simulink model "SEDC_Motor_model"  (R2021a)
settings: Solver=VariableStepAuto  StartTime=0.0  StopTime=inf  MaxStep=1e-3  RelTol=1e-3
values from neighbouring files (symbols this model uses):
  B = 0.01    [SEDC_Motor_model_int.m]
  J = 5    [SEDC_Motor_model_int.m]
  Kphi = 1.6    [SEDC_Motor_model_int.m]
  La = 0.1    [SEDC_Motor_model_int.m]
  Ra = 0.5    [SEDC_Motor_model_int.m]
  TL = 20    [SEDC_Motor_model_int.m]
  Va = 160    [SEDC_Motor_model_int.m]
settings Model: Creator=lenovo  LastModifiedBy=lenovo

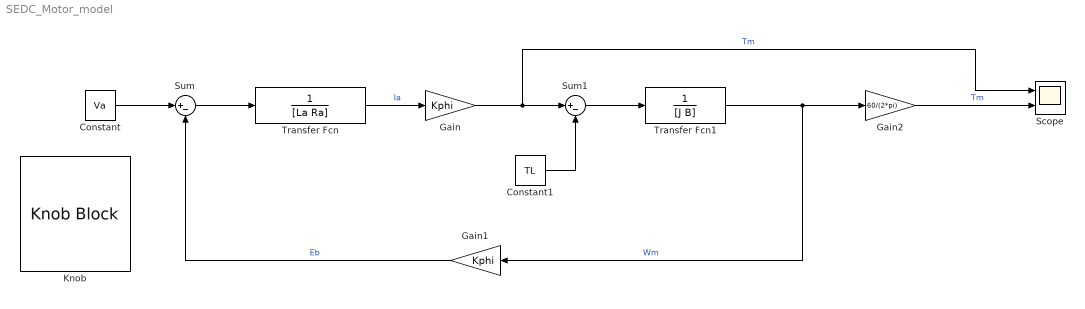
== system SEDC_Motor_model ==
  Constant : Constant  Value=Va
  Constant1 : Constant  Value=TL
  Gain : Gain  Gain=Kphi
  Gain1 : Gain  Gain=Kphi
  Gain2 : Gain  Gain=60/(2*pi)
  Knob : KnobBlock
  Scope : Scope  NumInputPorts=2
  Sum : Sum  Inputs=|+-
  Sum1 : Sum  Inputs=|+-
  Transfer Fcn : TransferFcn  Numerator=[1 ]  Denominator=[La Ra]
  Transfer Fcn1 : TransferFcn  Numerator=[1 ]  Denominator=[J B]
  wires:
  Constant/1 -> Sum/1
  Gain1/1 -> Sum/2  "Eb"
  Sum/1 -> Transfer Fcn/1
  Transfer Fcn/1 -> Gain/1  "Ia"
  Gain/1 -> Scope/1, Sum1/1  "Tm"
  Constant1/1 -> Sum1/2
  Sum1/1 -> Transfer Fcn1/1
  Transfer Fcn1/1 -> Gain1/1, Gain2/1  "Wm"
  Gain2/1 -> Scope/2  "Tm"
